simulink model "Ejercicio6_sim_sinOBS"  (R2020a)
settings: Solver=VariableStepAuto  StartTime=0.0  StopTime=10.0  RelTol=1e-3
values from neighbouring files (symbols this model uses):
  A = [[0 1 0 0 0];[-(cw+cs)/mw -ds/mw cs/mw ds/mw -1/mw];[0 0 0 1 0];[cs/mc ds/mc -cs/mc -ds/mc 1/mc];[0 0 0 0 -1/tau]]    [active_suspension_ctrl_design.m]
  B = [0 0 0 0 1/tau]'    [active_suspension_ctrl_design.m]
  C = [[-1 0 1 0 0];[cs/mc ds/mc -cs/mc -ds/mc 1/mc]]    [active_suspension_ctrl_design.m]
undefined symbols (not defined in the file or in its folder): K, kr
settings Model: Creator=juan  LastModifiedBy=juan

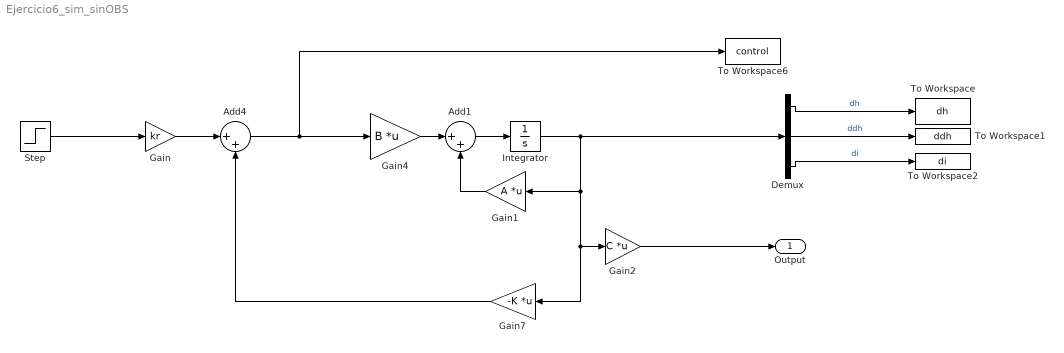
== system Ejercicio6_sim_sinOBS ==
  Add1 : Sum  Inputs=|++
  Add4 : Sum  Inputs=|++
  Demux : Demux  Outputs=3
  Gain : Gain  Gain=kr
  Gain1 : Gain  Gain=A  Multiplication=Matrix(K*u)
  Gain2 : Gain  Gain=C  Multiplication=Matrix(K*u)
  Gain4 : Gain  Gain=B  Multiplication=Matrix(K*u)
  Gain7 : Gain  Gain=-K  Multiplication=Matrix(K*u)
  Integrator : Integrator
  Step : Step  SampleTime=0
  To Workspace : ToWorkspace  VariableName=dh  SaveFormat=Structure With Time  SampleTime=-1
  To Workspace1 : ToWorkspace  VariableName=ddh  SaveFormat=Structure With Time  SampleTime=-1
  To Workspace2 : ToWorkspace  VariableName=di  SaveFormat=Structure With Time  SampleTime=-1
  To Workspace6 : ToWorkspace  VariableName=control  SaveFormat=Structure With Time  SampleTime=-1
  Output : Outport
  wires:
  Step/1 -> Gain/1
  Gain2/1 -> Output/1
  Add4/1 -> To Workspace6/1, Gain4/1
  Gain7/1 -> Add4/2
  Demux/2 -> To Workspace1/1  "ddh"
  Demux/1 -> To Workspace/1  "dh"
  Demux/3 -> To Workspace2/1  "di"
  Integrator/1 -> Gain7/1, Gain2/1, Gain1/1, Demux/1
  Gain1/1 -> Add1/2
  Gain/1 -> Add4/1
  Gain4/1 -> Add1/1
  Add1/1 -> Integrator/1
